simulink model "func5_a"  (R2020a)
settings: Solver=VariableStepAuto  StartTime=0.0  StopTime=10.0  RelTol=1e-3  EnableMultiTasking=on
undefined symbols (not defined in the file or in its folder): S, vsva2197, xcvc1902
libraries: ModelComposer x1, basics_5_lib x1
settings Model: Creator=abehbood  LastModifiedBy=viswanad
settings DataIOCC: ReturnWorkspaceOutputs=off
settings OptimizationCC: LifeSpan=inf
settings DebuggingCC: SFUnexpectedBacktrackingDiag=warning  SFNoUnconditionalDefaultTransitionDiag=warning  ArithmeticOperatorsInVariantConditions=warning
settings SFSimCC: SimUseLocalCustomCode=off  CustomCodeUndefinedFunction=UseInterfaceOnly
settings RTWCC: RTWUseLocalCustomCode=off
settings CodeAppCC: StateflowObjectComments=on
settings GRTTargetCC: TargetLangStandard=C89/C90 (ANSI)
settings ConfigComp: CovMetricSettings=dw  CovHtmlReporting=on  CovSaveCumulativeToWorkspaceVar=on  CovSaveSingleToWorkspaceVar=on  CovExternalEMLEnable=off

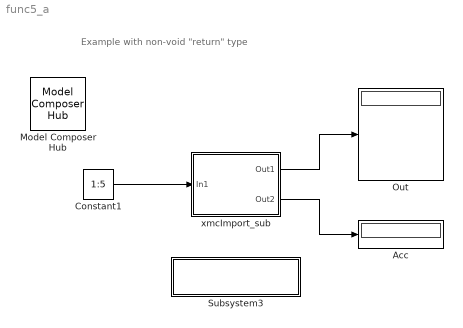
== system func5_a ==
  note: Example with non-void "return" type
  Acc : Display
  Constant1 : Constant  Value=1:5  OutDataTypeStr=int16  SampleTime=10
  Model Composer Hub : ModelComposer/Model Composer Hub  CodeGeneration=off  SubsystemName=xmcImport_sub  TargetDirectory=./code  ExportType=IP Catalog  IpVendor=xilinx.com  IpLibrary=hls  IpVersion=1.0  IpHWLanguage=Verilog  AieCompilerOptions={}  CreateTestbench=off  TestbenchStackSize=10  RunAieSim=off  AieSimTimeout=50000  RunAieSimProfiling=off  LaunchVitisAnalyzer=off  PlotOutput=off  RunX86Sim=off  X86SimTimeout=10  GenHwImage=off  PlatformType=Not Specified  ProjDevice=xcvc1902-vsva2197-2MP-e-S  ProjDevicePart=xcvc1902-vsva2197-2MP-e-S  SamplePeriod=-1  ClockFrequency=200  DataPathParallelism=1
  Out : Display
  Subsystem3 : Subsystem
      settings: OpenFcn=xmcOpenFileEx
      mask Display: disp(sprintf('Double Click to open\nthe main header file'))
  xmcImport_sub : Subsystem
  wires:
  Constant1/1 -> xmcImport_sub/1(In1)
  xmcImport_sub/1(Out1) -> Out/1
  xmcImport_sub/2(Out2) -> Acc/1

== system func5_a/Subsystem3 ==

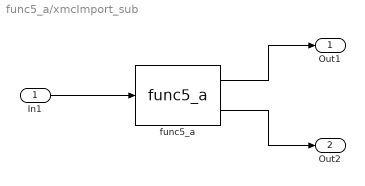
== system func5_a/xmcImport_sub ==
  In1 : Inport
  func5_a : basics_5_lib/func5_a  LibraryFunction=func5_a  IncludeFiles={'func5_a.h'}  SourceFiles={}  IncludeDirectories={}  TemplateParams={' '}  FunctionParamTypes={xmcDataType('int16_t'); xmcDataType('int16_t'); xmcDataType('int16_t')}  FunctionParamPassbys={0.000000000000000000e+00; 0.000000000000000000e+00; 0.000000000000000000e+00}  FunctionParamDimensions={'1'; '5'; '5'}  FunctionParamNames={'return'; 'in'; 'out'}  FunctionParamDir={2.000000000000000000e+00; 1.000000000000000000e+00; 2.000000000000000000e+00}  FunctionParamSupportsStreaming={false; false; false}  BufferDepth={'0'}  FunctionParamValues={'0'; '0'; '0'}
  Out1 : Outport
  Out2 : Outport  Port=2
  wires:
  func5_a/2 -> Out2/1
  In1/1 -> func5_a/1
  func5_a/1 -> Out1/1
